simulink model "BMS_Control_System"  (R2024b)
settings: Solver=VariableStepAuto  StartTime=0.0  StopTime=10.0  RelTol=1e-3
settings Model: Creator=pgoshomi  LastModifiedBy=pgoshomi

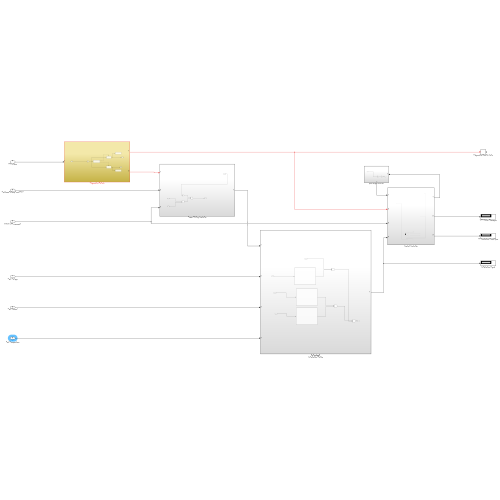
[thumbnail: Simulink's stored preview of the top-level diagram]
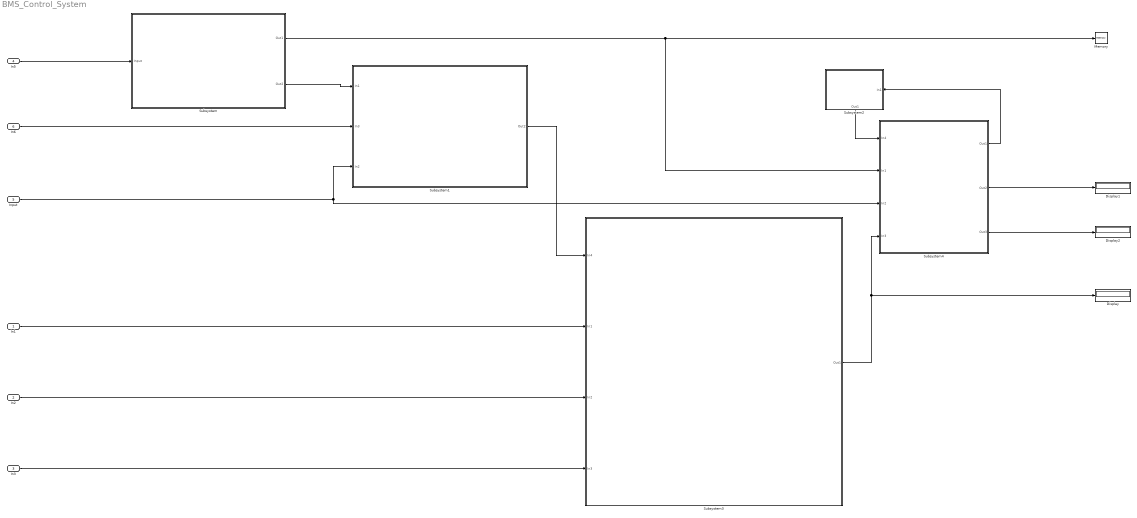
== system BMS_Control_System ==
  In1 : Inport  OutDataTypeStr=int8
      settings: AttributesFormatString=Pack Voltage
  In2 : Inport  Port=2
      settings: AttributesFormatString=Pack Current
  In3 : Inport  Port=3
      settings: AttributesFormatString=Pack Temperature
  In5 : Inport  Port=4
      settings: AttributesFormatString=HVIL status
  Input : Inport  Port=5
      settings: AttributesFormatString=EVCU CAN command
  In6 : Inport  Port=6
      settings: AttributesFormatString=HardwareWakeupFromEVCU
  Display : Display
      settings: AttributesFormatString=Initialization Signal
  Display1 : Display
      settings: AttributesFormatString=CAN Status Messages
  Display2 : Display
      settings: AttributesFormatString=HV Contactors Close/Open
  Memory : Memory
      settings: AttributesFormatString=Diagnostics/Trouble Code
  Subsystem : Subsystem
      settings: AttributesFormatString=Diagnostics Module
  Subsystem1 : Subsystem
      settings: AttributesFormatString=Power Moding Controller
  Subsystem2 : Subsystem
      settings: AttributesFormatString=prechargeController  PortSchema="{\"entries\":[{\"content\":{\"sides\":[{\"content\":{},\"type\":\"ConnectorPlacement.EquallySpacedRectSide\",\"uuid\":\"ab92245f-331b-4f4a-89ae-9b90f4abaae2\"},{\"content\":{\"connectorIds\":[\"In1\"],\"side\":\"RIGHT\"},\"type\":\"ConnectorPlacement.EquallySpacedRectSide\",\"uuid\":\"928ebfd6-5373-4512-94e5-162cfa91c5e4\"},{\"content\":{\"side\":\"TOP\"},\"type\":\"ConnectorPlacement.EquallySpacedRectSide\",\"uuid\":\"dc7d2ec8-a0b5-4d46-9e80-78af98197672\"},{\"content\":{\"connectorIds\":[\"Out1\"],\"side\":\"BOTTOM\"},\"type\":\"ConnectorPlacement.EquallySpacedRectSide\",\"uuid\":\"5f00ac33-258a-4d21-b1e0-e5a4b201fa67\"}]},\"type\":\"ConnectorPlacement.EquallySpacedConnector\",\"uuid\":\"5a2163c2-e595-4871-a7b7-df4990fbd52a\"}],\"packageUris\":[\"http://schema.mathworks.com/mf0/Connector/R2020b\"],\"version\":\"1.0\"}"
  Subsystem3 : Subsystem
      settings: AttributesFormatString=Initialisation Module
  Subsystem4 : Subsystem
      settings: AttributesFormatString=Contact Controller
  wires:
  In1/1 -> Subsystem3/2(In1)
  In2/1 -> Subsystem3/3(In2)
  In3/1 -> Subsystem3/4(In3)
  Subsystem/2(Out2) -> Subsystem1/1(In1)
  In6/1 -> Subsystem1/2(In3)
  Subsystem3/1(Out1) -> Subsystem4/4(In3), Display/1
  Subsystem1/1(Out2) -> Subsystem3/1(In4)
  Input/1 -> Subsystem1/3(In2), Subsystem4/3(In2)
  Subsystem/1(Out1) -> Memory/1, Subsystem4/2(In1)
  Subsystem2/1(Out1) -> Subsystem4/1(In4)
  Subsystem4/1(Out1) -> Subsystem2/1(In1)
  Subsystem4/2(Out2) -> Display1/1
  Subsystem4/3(Out3) -> Display2/1
  In5/1 -> Subsystem/1(Input)

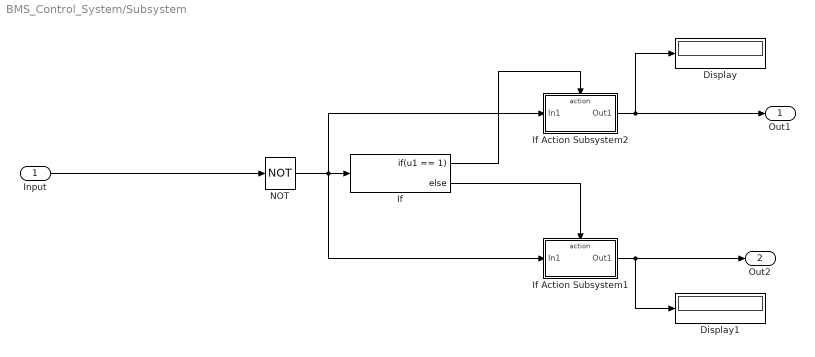
== system BMS_Control_System/Subsystem ==
  Input : Inport
  Display : Display
  Display1 : Display
  If : If  IfExpression=u1 == 1
  If Action Subsystem1 : Subsystem  TreatAsAtomicUnit=on
  If Action Subsystem2 : Subsystem  TreatAsAtomicUnit=on
  NOT : Logic  Operator=NOT  IconShape=distinctive  AllPortsSameDT=off  OutDataTypeStr=boolean
      settings: AttributesFormatString=Fault detector
  Out1 : Outport
  Out2 : Outport  Port=2
  wires:
  Input/1 -> NOT/1
  If/1 -> If Action Subsystem2/Action
  If/2 -> If Action Subsystem1/Action
  NOT/1 -> If/1, If Action Subsystem2/1(In1), If Action Subsystem1/1(In1)
  If Action Subsystem2/1(Out1) -> Display/1, Out1/1
  If Action Subsystem1/1(Out1) -> Display1/1, Out2/1

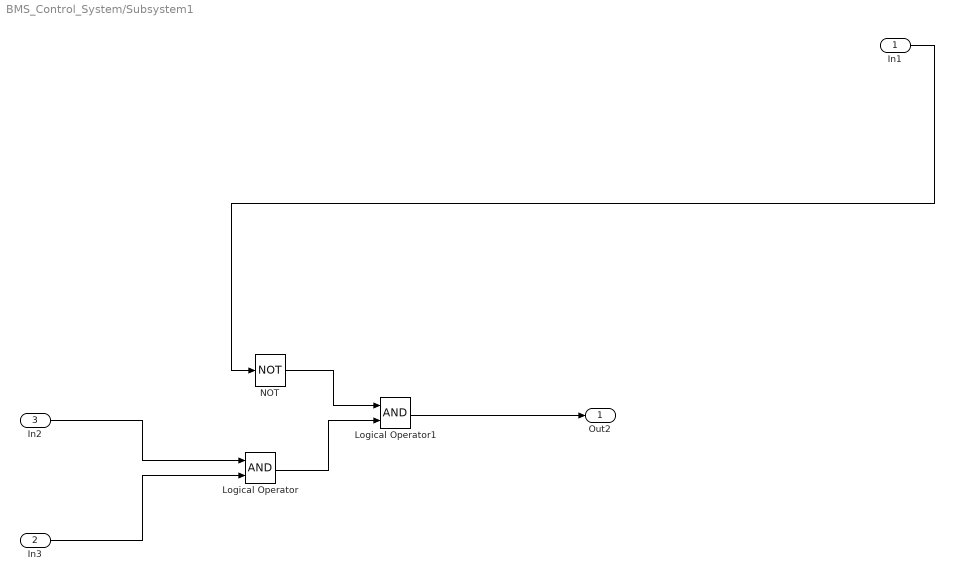
== system BMS_Control_System/Subsystem1 ==
  In1 : Inport
  In3 : Inport  Port=2
  In2 : Inport  Port=3
  Logical Operator : Logic  AllPortsSameDT=off  OutDataTypeStr=boolean
  Logical Operator1 : Logic  AllPortsSameDT=off  OutDataTypeStr=boolean
  NOT : Logic  Operator=NOT  IconShape=distinctive  AllPortsSameDT=off  OutDataTypeStr=boolean
  Out2 : Outport
  wires:
  In2/1 -> Logical Operator/1
  In3/1 -> Logical Operator/2
  Logical Operator1/1 -> Out2/1
  NOT/1 -> Logical Operator1/1
  In1/1 -> NOT/1
  Logical Operator/1 -> Logical Operator1/2

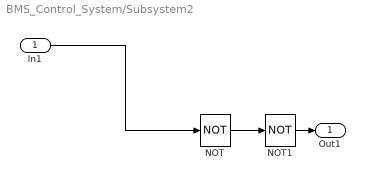
== system BMS_Control_System/Subsystem2 ==
  In1 : Inport
  NOT : Logic  Operator=NOT  IconShape=distinctive  AllPortsSameDT=off  OutDataTypeStr=boolean
  NOT1 : Logic  Operator=NOT  IconShape=distinctive  AllPortsSameDT=off  OutDataTypeStr=boolean
  Out1 : Outport
  wires:
  NOT1/1 -> Out1/1
  In1/1 -> NOT/1
  NOT/1 -> NOT1/1

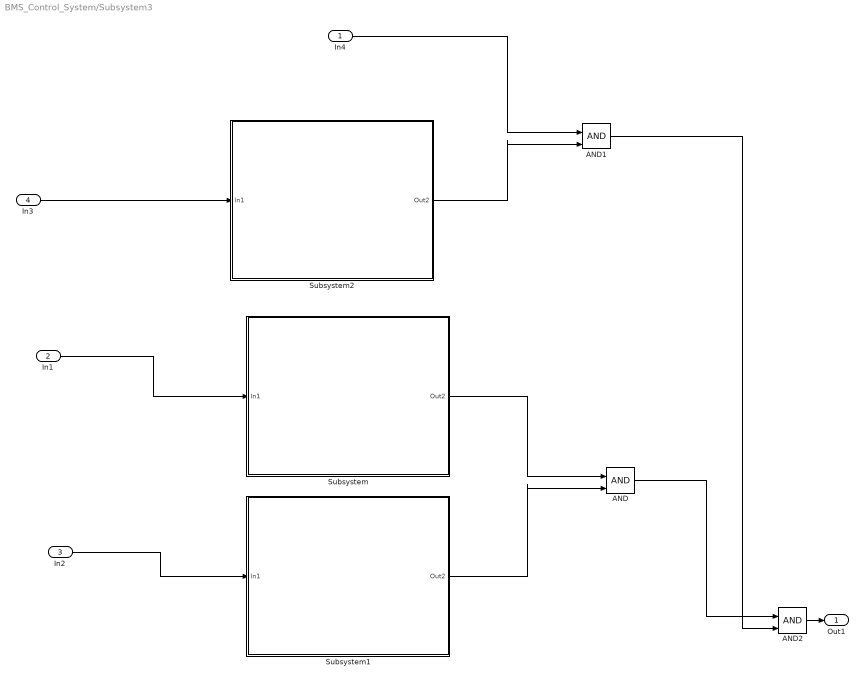
== system BMS_Control_System/Subsystem3 ==
  In4 : Inport
  In1 : Inport  Port=2
  In2 : Inport  Port=3
  In3 : Inport  Port=4
  AND : Logic  IconShape=distinctive  AllPortsSameDT=off  OutDataTypeStr=boolean
  AND1 : Logic  IconShape=distinctive  AllPortsSameDT=off  OutDataTypeStr=boolean
  AND2 : Logic  IconShape=distinctive  AllPortsSameDT=off  OutDataTypeStr=boolean
  Subsystem : Subsystem  Description=Voltage Validator
      settings: AttributesFormatString=Voltage Validator
  Subsystem1 : Subsystem
      settings: AttributesFormatString=Current Validator
  Subsystem2 : Subsystem
      settings: AttributesFormatString=Temparature Validator
  Out1 : Outport
  wires:
  AND2/1 -> Out1/1
  In2/1 -> Subsystem1/1(In1)
  AND/1 -> AND2/1
  Subsystem2/1(Out2) -> AND1/2
  Subsystem1/1(Out2) -> AND/2
  Subsystem/1(Out2) -> AND/1
  In1/1 -> Subsystem/1(In1)
  In3/1 -> Subsystem2/1(In1)
  AND1/1 -> AND2/2
  In4/1 -> AND1/1

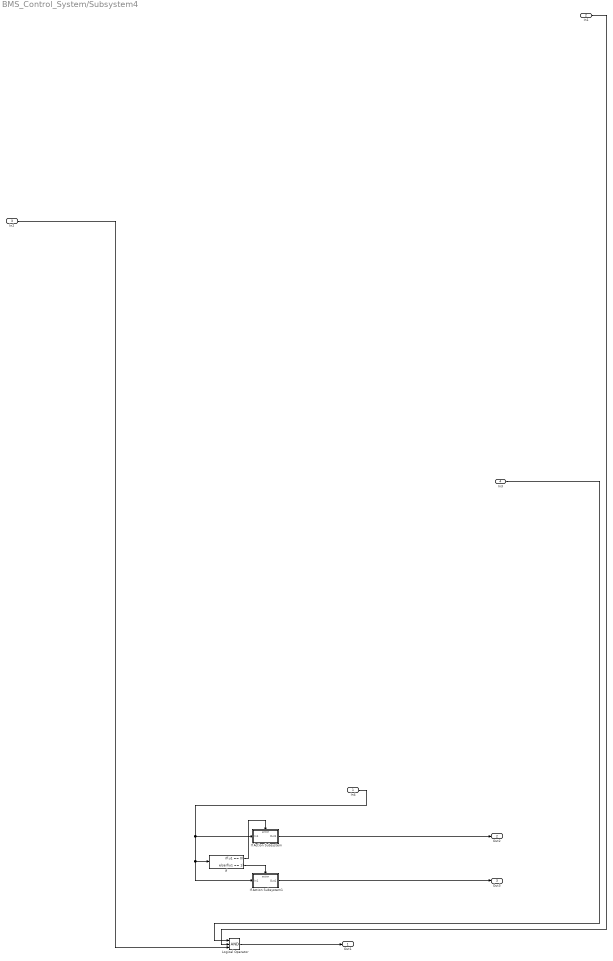
== system BMS_Control_System/Subsystem4 ==
  In4 : Inport
  In1 : Inport  Port=2
  In2 : Inport  Port=3
  In3 : Inport  Port=4
  If : If  IfExpression=u1 == 0  ElseIfExpressions=u1 == 1  ShowElse=off
  If Action Subsystem : Subsystem  TreatAsAtomicUnit=on
  If Action Subsystem1 : Subsystem  TreatAsAtomicUnit=on
  Logical Operator : Logic  Inputs=3  AllPortsSameDT=off  OutDataTypeStr=boolean
  Out1 : Outport
  Out2 : Outport  Port=2
  Out3 : Outport  Port=3
  wires:
  In2/1 -> Logical Operator/3
  In3/1 -> Logical Operator/1
  Logical Operator/1 -> Out1/1
  In1/1 -> Logical Operator/2
  If/1 -> If Action Subsystem/Action
  If Action Subsystem/1(Out1) -> Out2/1
  If/2 -> If Action Subsystem1/Action
  In4/1 -> If Action Subsystem1/1(In1), If/1, If Action Subsystem/1(In1)
  If Action Subsystem1/1(Out1) -> Out3/1

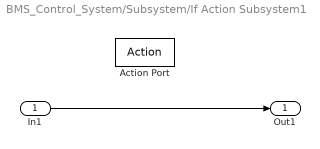
== system BMS_Control_System/Subsystem/If Action Subsystem1 ==
  In1 : Inport
  Action Port : ActionPort  ActionPortLabel=else
  Out1 : Outport
  wires:
  In1/1 -> Out1/1

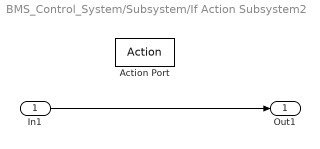
== system BMS_Control_System/Subsystem/If Action Subsystem2 ==
  In1 : Inport
  Action Port : ActionPort  ActionPortLabel=if(u1 == 1)
  Out1 : Outport
  wires:
  In1/1 -> Out1/1

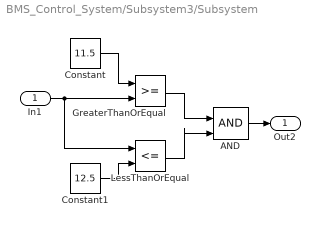
== system BMS_Control_System/Subsystem3/Subsystem ==
  In1 : Inport
  AND : Logic  Description=Validate if a value is in between a specified range  IconShape=distinctive  AllPortsSameDT=off  OutDataTypeStr=boolean
  Constant : Constant  Value=11.5
      settings: AttributesFormatString=lowerThreshold
  Constant1 : Constant  Value=12.5
      settings: AttributesFormatString=upperThreshold
  GreaterThanOrEqual : RelationalOperator  OutDataTypeStr=boolean  RndMeth=Simplest  InputSameDT=off
  LessThanOrEqual : RelationalOperator  Operator=<=  OutDataTypeStr=boolean  RndMeth=Simplest  InputSameDT=off
  Out2 : Outport  Description=Voltage Validator
  wires:
  AND/1 -> Out2/1
  GreaterThanOrEqual/1 -> AND/1
  LessThanOrEqual/1 -> AND/2
  In1/1 -> GreaterThanOrEqual/2, LessThanOrEqual/1
  Constant1/1 -> LessThanOrEqual/2
  Constant/1 -> GreaterThanOrEqual/1

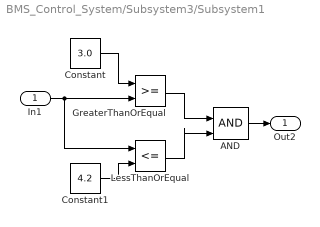
== system BMS_Control_System/Subsystem3/Subsystem1 ==
  In1 : Inport
  AND : Logic  Description=Validate if a value is in between a specified range  IconShape=distinctive  AllPortsSameDT=off  OutDataTypeStr=boolean
  Constant : Constant  Value=3.0
      settings: AttributesFormatString=lowerThreshold
  Constant1 : Constant  Value=4.2
      settings: AttributesFormatString=upperThreshold
  GreaterThanOrEqual : RelationalOperator  OutDataTypeStr=boolean  RndMeth=Simplest  InputSameDT=off
  LessThanOrEqual : RelationalOperator  Operator=<=  OutDataTypeStr=boolean  RndMeth=Simplest  InputSameDT=off
  Out2 : Outport  Description=Voltage Validator
  wires:
  AND/1 -> Out2/1
  GreaterThanOrEqual/1 -> AND/1
  LessThanOrEqual/1 -> AND/2
  In1/1 -> GreaterThanOrEqual/2, LessThanOrEqual/1
  Constant1/1 -> LessThanOrEqual/2
  Constant/1 -> GreaterThanOrEqual/1

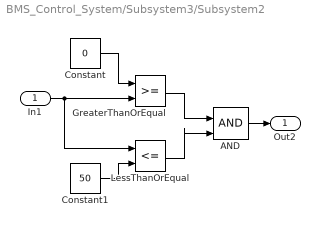
== system BMS_Control_System/Subsystem3/Subsystem2 ==
  In1 : Inport
  AND : Logic  Description=Validate if a value is in between a specified range  IconShape=distinctive  AllPortsSameDT=off  OutDataTypeStr=boolean
  Constant : Constant  Value=0
      settings: AttributesFormatString=lowerThreshold
  Constant1 : Constant  Value=50
      settings: AttributesFormatString=upperThreshold
  GreaterThanOrEqual : RelationalOperator  OutDataTypeStr=boolean  RndMeth=Simplest  InputSameDT=off
  LessThanOrEqual : RelationalOperator  Operator=<=  OutDataTypeStr=boolean  RndMeth=Simplest  InputSameDT=off
  Out2 : Outport  Description=Voltage Validator
  wires:
  AND/1 -> Out2/1
  GreaterThanOrEqual/1 -> AND/1
  LessThanOrEqual/1 -> AND/2
  In1/1 -> GreaterThanOrEqual/2, LessThanOrEqual/1
  Constant1/1 -> LessThanOrEqual/2
  Constant/1 -> GreaterThanOrEqual/1

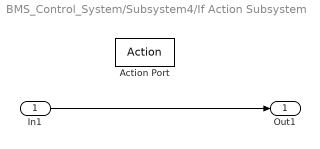
== system BMS_Control_System/Subsystem4/If Action Subsystem ==
  In1 : Inport
  Action Port : ActionPort  ActionPortLabel=if(u1 == 0)
  Out1 : Outport
  wires:
  In1/1 -> Out1/1

== system BMS_Control_System/Subsystem4/If Action Subsystem1 ==
  In1 : Inport
  Action Port : ActionPort  ActionPortLabel=elseif(u1 == 1)
  Out1 : Outport
  wires:
  In1/1 -> Out1/1
